simulink model "ddc_bpm_476_066"  (Simulink 7.8)
settings: Solver=ode45  StartTime=0.0  StopTime=2e-3  RelTol=1e-3
undefined symbols (not defined in the file): decim_factor_poly_35, dt_sim, frev_476, Fs_adc, n_ch, n_ovs, R_fofb, R_sec, R_sec_cfir, R_sec_pfir, R_tbt, xlipgetpartsetting
libraries: xbsIndex_r4 x1408, simulink x7
(part 9 of 11)

== system ddc_bpm_476_066/TBT_amp/TBT_amp0/TBT_poly_decim ==
  Q_in : Inport
  I_in : Inport  Port=2
  ch_in : Inport  Port=3
  Register1 : xbsIndex_r4/Register  init=0  rst=off  en=on  dbl_ovrd=off  block_type=register
  Register2 : xbsIndex_r4/Register  init=0  rst=off  en=off  dbl_ovrd=off  block_type=register
  Register3 : xbsIndex_r4/Register  init=0  rst=off  en=on  dbl_ovrd=off  block_type=register
  Register6 : xbsIndex_r4/Register  init=0  rst=off  en=off  dbl_ovrd=off  block_type=register
  Reinterpret : xbsIndex_r4/Reinterpret  force_arith_type=on  arith_type="Signed  (2's comp)"  force_bin_pt=on  bin_pt=23  block_type=reinterpret
      settings: block_version=10.1
  Reinterpret1 : xbsIndex_r4/Reinterpret  force_arith_type=on  arith_type="Signed  (2's comp)"  force_bin_pt=on  bin_pt=23  block_type=reinterpret
      settings: block_version=10.1
  ST3 : Subsystem
  Scope : Scope
      settings: YMin=1  YMax=1  SaveName=ScopeData4
  TBT_poly : xbsIndex_r4/FIR Compiler 6.3   coefficientvector=Hpoly_35.Numerator  coefficient_sets=1  coefficient_reload=off  filter_type=Decimation  rate_change_type=Integer  interpolation_rate=1  decimation_rate=decim_factor_poly_35  zero_pack_factor=1  channel_sequence=Basic  number_channels=2  pattern_list='P4-0,P4-1,P4-2,P4-3,P4-4'  number_paths=2  ratespecification=Maximum_Possible  sampleperiod=1  hardwareoversamplingrate=1  coefficient_sign=Signed  quantization=Quantize_Only  coefficient_width=16  bestprecision=on  coefficient_fractional_bits=20  coefficient_structure=Inferred  output_rounding_mode=Convergent_Rounding_to_Even  output_width=25  filter_architecture=Systolic_Multiply_Accumulate  optimization_goal=Area  data_buffer_type=Automatic  coefficient_buffer_type=Automatic  input_buffer_type=Automatic  output_buffer_type=Automatic  preference_for_other_storage=Automatic  multi_column_support=Automatic  columnconfig='13'  inter_column_pipe_length=4  data_has_tlast=Not_Required  m_data_has_tready=off  s_data_has_fifo=off  s_data_has_tuser=Chan_ID_Field  m_data_has_tuser=Chan_ID_Field  s_config_sync_mode=On_Vector  s_config_method=Single  num_reload_slots=1  has_aclken=off  has_aresetn=off  infoeditControl=ARESETn must be asserted for a minmum of 2 cycles  trim_axipin_name=on  passband_min=0.0  passband_max=0.5  stopband_min=0.5  stopband_max=1.0  filter_selection=1  gui_behaviour=Sysgen_GUI  data_sign=Signed  data_width=16  data_fractional_bits=0  data_tuser_width=1  wrapper_available=true  ip_wrap_arbitrary_binary_point=true  simulation_type=external_xfix  simulation_model=firv6_3_CModel:firv6_3_cmodel  ip_name=FIR Compiler  ip_version=6.3  dsptool_ready=true  ipcore_usecache=true  ipcore_useipmodelcache=true  ipcore_xco_need_fpga_part=true  port_translation_map={ 'aclken' => 'en', 'aresetn' => 'rst' }  run_core_at_system_period=true  ipcore_fpga_part=xlipgetpartsetting(gcb, {'virtex6', 'xc6vlx75t', '-3', 'ff784'})  block_type=fir_compiler_v6_3
      settings: infoedit=Maximum Possible : Maximizes oversampling rate. Abstracted input handshake (no s_data_tvalid) and automatic rate propagation.<br>Hardware Oversampling Rate : Specifies oversampling rate relative to the input sample period. Abstracted input handshake (no s_data_tvalid) and automatic rate propagation.<br>Sample Period : Specifies absolute oversampling rate. No input handshake abstraction (exposes s_data_tvalid) and no rate propagation.
  TDDM_TBT : Subsystem
  Terminator : Terminator
  Trunc : Subsystem
  Trunc1 : Subsystem
  tbt_decim_ch01_incorrect_o : xbsIndex_r4/Gateway Out  inherit_from_input=on  hdl_port=on  timing_constraint=Data Rate  locs_specified=off  LOCs={}  UseAsDAC=off  DACChannel='1'  block_type=gatewayout
      settings: infoedit="Gateway out block.  Converts Xilinx fixed-point or floating-point type inputs into ouputs of type Simulink integer, single, double, or fixed point.<br><br>Hardware notes:  In hardware these blocks become top level output ports or are discarded, depending on how they are configured."
  tbt_decim_ch0_i_o : xbsIndex_r4/Gateway Out  inherit_from_input=on  hdl_port=on  timing_constraint=Data Rate  locs_specified=off  LOCs={}  UseAsDAC=off  DACChannel='1'  block_type=gatewayout
      settings: infoedit="Gateway out block.  Converts Xilinx fixed-point or floating-point type inputs into ouputs of type Simulink integer, single, double, or fixed point.<br><br>Hardware notes:  In hardware these blocks become top level output ports or are discarded, depending on how they are configured."
  tbt_decim_ch0_q_o : xbsIndex_r4/Gateway Out  inherit_from_input=on  hdl_port=on  timing_constraint=Data Rate  locs_specified=off  LOCs={}  UseAsDAC=off  DACChannel='1'  block_type=gatewayout
      settings: infoedit="Gateway out block.  Converts Xilinx fixed-point or floating-point type inputs into ouputs of type Simulink integer, single, double, or fixed point.<br><br>Hardware notes:  In hardware these blocks become top level output ports or are discarded, depending on how they are configured."
  tbt_decim_ch1_i_o : xbsIndex_r4/Gateway Out  inherit_from_input=on  hdl_port=on  timing_constraint=Data Rate  locs_specified=off  LOCs={}  UseAsDAC=off  DACChannel='1'  block_type=gatewayout
      settings: infoedit="Gateway out block.  Converts Xilinx fixed-point or floating-point type inputs into ouputs of type Simulink integer, single, double, or fixed point.<br><br>Hardware notes:  In hardware these blocks become top level output ports or are discarded, depending on how they are configured."
  tbt_decim_ch1_q_o : xbsIndex_r4/Gateway Out  inherit_from_input=on  hdl_port=on  timing_constraint=Data Rate  locs_specified=off  LOCs={}  UseAsDAC=off  DACChannel='1'  block_type=gatewayout
      settings: infoedit="Gateway out block.  Converts Xilinx fixed-point or floating-point type inputs into ouputs of type Simulink integer, single, double, or fixed point.<br><br>Hardware notes:  In hardware these blocks become top level output ports or are discarded, depending on how they are configured."
  tbt_poly_i_scope : Scope  NumInputPorts=2
      settings: TimeRange=0.00011214  YMin=-0.1~-1.5  YMax=1~1.5  SaveName=ScopeData15  MaxDataPoints=1000000  SampleInput=on
  tbt_poly_q_scope : Scope  NumInputPorts=2
      settings: TimeRange=0.00011214  YMin=0.00109935~-0.000380039  YMax=0.00109935~-0.000380039  SaveName=ScopeData18  MaxDataPoints=1000000  SampleInput=on
  Q_out : Outport
  I_out : Outport  Port=2
  valid_out : Outport  Port=3
  ch_out : Outport  Port=4
  wires:
  Q_in/1 -> TBT_poly/2
  TBT_poly/4 -> Reinterpret/1
  TBT_poly/5 -> Reinterpret1/1
  I_in/1 -> TBT_poly/3
  TBT_poly/1 -> Terminator/1
  TBT_poly/3 -> Register2/1
  ch_in/1 -> ST3/1(In), TBT_poly/1
  [tbt_poly_q_out] -> Trunc/1(din)
  [tbt_poly_ch_out] -> TDDM_TBT/3(tbt_ch_in)
  [tbt_poly_i_out] -> Trunc1/1(din)
  Trunc/1(dout) -> TDDM_TBT/1(tbt_q_in)
  Trunc1/1(dout) -> TDDM_TBT/2(tbt_i_in)
  tbt_decim_ch0_q_o/1 -> tbt_poly_q_scope/1
  tbt_decim_ch1_q_o/1 -> tbt_poly_q_scope/2
  TDDM_TBT/1(poly35_ch0_q_out) -> tbt_decim_ch0_q_o/1
  TDDM_TBT/2(poly35_ch1_q_out) -> tbt_decim_ch1_q_o/1
  tbt_decim_ch0_i_o/1 -> tbt_poly_i_scope/1
  tbt_decim_ch1_i_o/1 -> tbt_poly_i_scope/2
  TDDM_TBT/3(poly35_ch0_i_out) -> tbt_decim_ch0_i_o/1
  TDDM_TBT/4(poly35_ch1_i_out) -> tbt_decim_ch1_i_o/1
  Register2/1 -> ch_out/1, [tbt_poly_ch_out]
  TBT_poly/2 -> Register6/1, Register1/2, Register3/2
  Register6/1 -> valid_out/1
  Reinterpret/1 -> Register1/1
  Register1/1 -> Q_out/1, [tbt_poly_q_out]
  Register3/1 -> I_out/1, [tbt_poly_i_out]
  Reinterpret1/1 -> Register3/1
  tbt_decim_ch01_incorrect_o/1 -> Scope/1
  TBT_poly/6 -> tbt_decim_ch01_incorrect_o/1

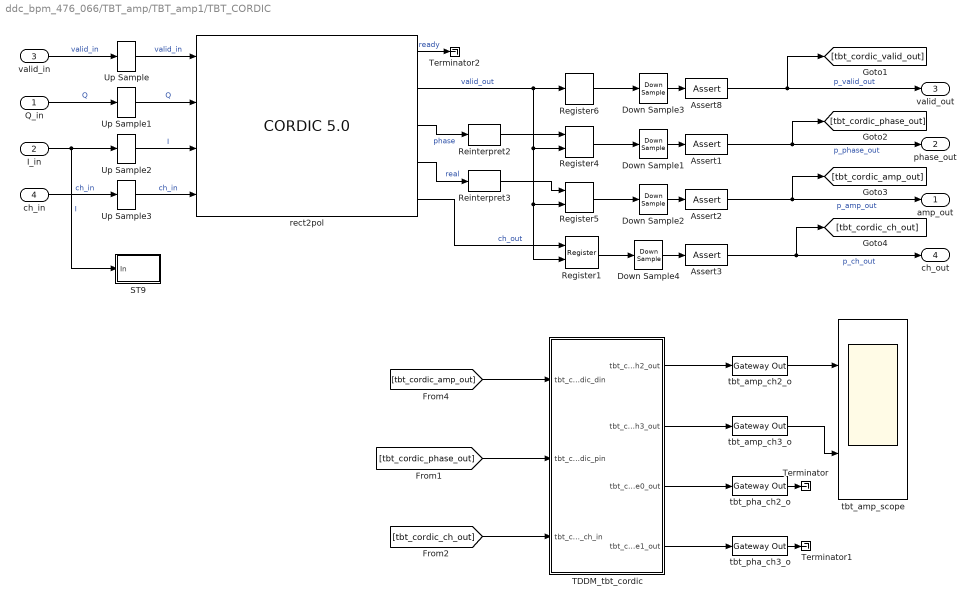
== system ddc_bpm_476_066/TBT_amp/TBT_amp1/TBT_CORDIC ==
  Q_in : Inport
  I_in : Inport  Port=2
  valid_in : Inport  Port=3
  ch_in : Inport  Port=4
  Assert{1..3,8} (4 alike) : xbsIndex_r4/Assert  assert_type=off  type_source=Explicitly  gui_display_data_type=Fixed-point  arith_type="Signed  (2's comp)"  n_bits=16  bin_pt=14  preci_type=Single  exp_width=8  frac_width=24  assert_rate=on  rate_source=Explicitly  period=(1/Fs_adc/n_ovs)*decim_factor_poly_35  output_port=on  block_type=assert
  Down Sample{1..4} (4 alike) : xbsIndex_r4/Down Sample  sample_ratio=decim_factor_poly_35  sample_phase="Last Value of Frame  (most efficient)"  en=off  latency=1  dbl_ovrd=off  block_type=dsamp
  Register1 : xbsIndex_r4/Register  init=0  rst=off  en=on  dbl_ovrd=off  block_type=register
  Register4 : xbsIndex_r4/Register  init=0  rst=off  en=on  dbl_ovrd=off  block_type=register
  Register5 : xbsIndex_r4/Register  init=0  rst=off  en=on  dbl_ovrd=off  block_type=register
  Register6 : xbsIndex_r4/Register  init=0  rst=off  en=off  dbl_ovrd=off  block_type=register
  Reinterpret2 : xbsIndex_r4/Reinterpret  force_arith_type=off  arith_type=Unsigned  force_bin_pt=off  bin_pt=18  block_type=reinterpret
  Reinterpret3 : xbsIndex_r4/Reinterpret  force_arith_type=off  arith_type=Unsigned  force_bin_pt=off  bin_pt=19  block_type=reinterpret
  ST9 : Subsystem
  TDDM_tbt_cordic : Subsystem
  Terminator : Terminator
  Terminator1 : Terminator
  Terminator2 : Terminator
  Up Sample : xbsIndex_r4/Up Sample  sample_ratio=R_tbt  copy_samples=off  en=off  latency=0  dbl_ovrd=off  block_type=usamp
  Up Sample1 : xbsIndex_r4/Up Sample  sample_ratio=R_tbt  copy_samples=on  en=off  latency=0  dbl_ovrd=off  block_type=usamp
  Up Sample2 : xbsIndex_r4/Up Sample  sample_ratio=R_tbt  copy_samples=on  en=off  latency=0  dbl_ovrd=off  block_type=usamp
  Up Sample3 : xbsIndex_r4/Up Sample  sample_ratio=R_tbt  copy_samples=on  en=off  latency=0  dbl_ovrd=off  block_type=usamp
  rect2pol : xbsIndex_r4/CORDIC 5.0   functional_selection=Translate  architectural_configuration=Word_Serial  pipelining_mode=Optimal  data_format=SignedFraction  phase_format=Radians  input_width=25  output_width=24  round_mode=Nearest_Even  iterations=0  precision=0  compensation_scaling=Embedded_Multiplier  coarse_rotation=on  aclken=off  aresetn=off  out_tready=off  cartesian_has_tuser=on  cartesian_has_tlast=off  cartesian_tuser_width=1  phase_has_tuser=off  phase_has_tlast=off  phase_tuser_width=1  out_tlast_behv=Null  flow_control=NonBlocking  optimize_goal=Resources  trim_axipin_name=on  ip_name=CORDIC  ip_version=5.0  dsptool_ready=true  ipcore_usecache=true  ipcore_useipmodelcache=true  wrapper_available=true  port_translation_map={ 'aclken' => 'en', 'aresetn' => 'rst' }  block_type=cordic_v5_0
      settings: infoedit=CORDIC 5.0
  tbt_amp_ch2_o : xbsIndex_r4/Gateway Out  inherit_from_input=on  hdl_port=on  timing_constraint=Data Rate  locs_specified=off  LOCs={}  UseAsDAC=off  DACChannel='1'  block_type=gatewayout
      settings: infoedit="Gateway out block.  Converts Xilinx fixed-point or floating-point type inputs into ouputs of type Simulink integer, single, double, or fixed point.<br><br>Hardware notes:  In hardware these blocks become top level output ports or are discarded, depending on how they are configured."
  tbt_amp_ch3_o : xbsIndex_r4/Gateway Out  inherit_from_input=on  hdl_port=on  timing_constraint=Data Rate  locs_specified=off  LOCs={}  UseAsDAC=off  DACChannel='1'  block_type=gatewayout
      settings: infoedit="Gateway out block.  Converts Xilinx fixed-point or floating-point type inputs into ouputs of type Simulink integer, single, double, or fixed point.<br><br>Hardware notes:  In hardware these blocks become top level output ports or are discarded, depending on how they are configured."
  tbt_amp_scope : Scope  NumInputPorts=2
      settings: TimeRange=0.00011214  YMin=0.109899~0.0274758  YMax=0.109899~0.0274758  SaveName=ScopeData19  MaxDataPoints=1000000  SampleInput=on
  tbt_pha_ch2_o : xbsIndex_r4/Gateway Out  inherit_from_input=on  hdl_port=on  timing_constraint=Data Rate  locs_specified=off  LOCs={}  UseAsDAC=off  DACChannel='1'  block_type=gatewayout
      settings: infoedit="Gateway out block.  Converts Xilinx fixed-point or floating-point type inputs into ouputs of type Simulink integer, single, double, or fixed point.<br><br>Hardware notes:  In hardware these blocks become top level output ports or are discarded, depending on how they are configured."
  tbt_pha_ch3_o : xbsIndex_r4/Gateway Out  inherit_from_input=off  hdl_port=on  timing_constraint=Data Rate  locs_specified=off  LOCs={}  UseAsDAC=off  DACChannel='1'  block_type=gatewayout
      settings: infoedit="Gateway out block.  Converts Xilinx fixed-point or floating-point type inputs into ouputs of type Simulink integer, single, double, or fixed point.<br><br>Hardware notes:  In hardware these blocks become top level output ports or are discarded, depending on how they are configured."
  amp_out : Outport
  phase_out : Outport  Port=2
  valid_out : Outport  Port=3
  ch_out : Outport  Port=4
  wires:
  [tbt_cordic_amp_out] -> TDDM_tbt_cordic/1(tbt_cordic_din)
  [tbt_cordic_ch_out] -> TDDM_tbt_cordic/3(tbt_cordic_ch_in)
  tbt_amp_ch2_o/1 -> tbt_amp_scope/1
  tbt_amp_ch3_o/1 -> tbt_amp_scope/2
  TDDM_tbt_cordic/1(tbt_cordic_ch2_out) -> tbt_amp_ch2_o/1
  TDDM_tbt_cordic/2(tbt_cordic_ch3_out) -> tbt_amp_ch3_o/1
  TDDM_tbt_cordic/3(tbt_cordic_phase0_out) -> tbt_pha_ch2_o/1
  TDDM_tbt_cordic/4(tbt_cordic_phase1_out) -> tbt_pha_ch3_o/1
  tbt_pha_ch2_o/1 -> Terminator/1
  tbt_pha_ch3_o/1 -> Terminator1/1
  [tbt_cordic_phase_out] -> TDDM_tbt_cordic/2(tbt_cordic_pin)
  Register4/1 -> Down Sample1/1
  Register5/1 -> Down Sample2/1
  Register6/1 -> Down Sample3/1
  Reinterpret2/1 -> Register4/1
  Reinterpret3/1 -> Register5/1
  valid_in/1 -> Up Sample/1  "valid_in"
  Q_in/1 -> Up Sample1/1  "Q"
  I_in/1 -> ST9/1(In), Up Sample2/1  "I"
  ch_in/1 -> Up Sample3/1  "ch_in"
  Register1/1 -> Down Sample4/1
  rect2pol/2 -> Register6/1, Register4/2, Register5/2, Register1/2  "valid_out"
  rect2pol/3 -> Reinterpret2/1  "phase"
  rect2pol/4 -> Reinterpret3/1  "real"
  rect2pol/5 -> Register1/1  "ch_out"
  rect2pol/1 -> Terminator2/1  "ready"
  Up Sample/1 -> rect2pol/1  "valid_in"
  Up Sample1/1 -> rect2pol/2  "Q"
  Up Sample2/1 -> rect2pol/3  "I"
  Up Sample3/1 -> rect2pol/4  "ch_in"
  Down Sample3/1 -> Assert8/1
  Assert8/1 -> valid_out/1, [tbt_cordic_valid_out]  "p_valid_out"
  Down Sample1/1 -> Assert1/1
  Down Sample2/1 -> Assert2/1
  Down Sample4/1 -> Assert3/1
  Assert1/1 -> phase_out/1, [tbt_cordic_phase_out]  "p_phase_out"
  Assert2/1 -> amp_out/1, [tbt_cordic_amp_out]  "p_amp_out"
  Assert3/1 -> ch_out/1, [tbt_cordic_ch_out]  "p_ch_out"

== system ddc_bpm_476_066/TBT_amp/TBT_amp1/TBT_poly_decim ==
  note: Introduced delays to avoid incorrect signal on the output
  Q_in : Inport
  I_in : Inport  Port=2
  ch_in : Inport  Port=3
  Register1 : xbsIndex_r4/Register  init=0  rst=off  en=on  dbl_ovrd=off  block_type=register
  Register2 : xbsIndex_r4/Register  init=0  rst=off  en=off  dbl_ovrd=off  block_type=register
  Register3 : xbsIndex_r4/Register  init=0  rst=off  en=on  dbl_ovrd=off  block_type=register
  Register6 : xbsIndex_r4/Register  init=0  rst=off  en=off  dbl_ovrd=off  block_type=register
  Reinterpret : xbsIndex_r4/Reinterpret  force_arith_type=on  arith_type="Signed  (2's comp)"  force_bin_pt=on  bin_pt=23  block_type=reinterpret
      settings: block_version=10.1
  Reinterpret1 : xbsIndex_r4/Reinterpret  force_arith_type=on  arith_type="Signed  (2's comp)"  force_bin_pt=on  bin_pt=23  block_type=reinterpret
      settings: block_version=10.1
  Scope : Scope
      settings: YMin=0.95  YMax=1.05  SaveName=ScopeData5
  TBT_poly : xbsIndex_r4/FIR Compiler 6.3   coefficientvector=Hpoly_35.Numerator  coefficient_sets=1  coefficient_reload=off  filter_type=Decimation  rate_change_type=Integer  interpolation_rate=1  decimation_rate=decim_factor_poly_35  zero_pack_factor=1  channel_sequence=Basic  number_channels=2  pattern_list='P4-0,P4-1,P4-2,P4-3,P4-4'  number_paths=2  ratespecification=Maximum_Possible  sampleperiod=1  hardwareoversamplingrate=2  coefficient_sign=Signed  quantization=Quantize_Only  coefficient_width=16  bestprecision=on  coefficient_fractional_bits=20  coefficient_structure=Inferred  output_rounding_mode=Convergent_Rounding_to_Even  output_width=25  filter_architecture=Systolic_Multiply_Accumulate  optimization_goal=Area  data_buffer_type=Automatic  coefficient_buffer_type=Automatic  input_buffer_type=Automatic  output_buffer_type=Automatic  preference_for_other_storage=Automatic  multi_column_support=Automatic  columnconfig='13'  inter_column_pipe_length=4  data_has_tlast=Not_Required  m_data_has_tready=off  s_data_has_fifo=off  s_data_has_tuser=Chan_ID_Field  m_data_has_tuser=Chan_ID_Field  s_config_sync_mode=On_Vector  s_config_method=Single  num_reload_slots=1  has_aclken=off  has_aresetn=off  infoeditControl=ARESETn must be asserted for a minmum of 2 cycles  trim_axipin_name=on  passband_min=0.0  passband_max=0.5  stopband_min=0.5  stopband_max=1.0  filter_selection=1  gui_behaviour=Sysgen_GUI  data_sign=Signed  data_width=16  data_fractional_bits=0  data_tuser_width=1  wrapper_available=true  ip_wrap_arbitrary_binary_point=true  simulation_type=external_xfix  simulation_model=firv6_3_CModel:firv6_3_cmodel  ip_name=FIR Compiler  ip_version=6.3  dsptool_ready=true  ipcore_usecache=true  ipcore_useipmodelcache=true  ipcore_xco_need_fpga_part=true  port_translation_map={ 'aclken' => 'en', 'aresetn' => 'rst' }  run_core_at_system_period=true  ipcore_fpga_part=xlipgetpartsetting(gcb, {'virtex6', 'xc6vlx75t', '-3', 'ff784'})  block_type=fir_compiler_v6_3
      settings: infoedit=Maximum Possible : Maximizes oversampling rate. Abstracted input handshake (no s_data_tvalid) and automatic rate propagation.<br>Hardware Oversampling Rate : Specifies oversampling rate relative to the input sample period. Abstracted input handshake (no s_data_tvalid) and automatic rate propagation.<br>Sample Period : Specifies absolute oversampling rate. No input handshake abstraction (exposes s_data_tvalid) and no rate propagation.
  TDDM_TBT : Subsystem
  Terminator : Terminator
  Trunc : Subsystem
  Trunc1 : Subsystem
  tbt_decim_ch23_incorrect_o : xbsIndex_r4/Gateway Out  inherit_from_input=on  hdl_port=on  timing_constraint=Data Rate  locs_specified=off  LOCs={}  UseAsDAC=off  DACChannel='1'  block_type=gatewayout
      settings: infoedit="Gateway out block.  Converts Xilinx fixed-point or floating-point type inputs into ouputs of type Simulink integer, single, double, or fixed point.<br><br>Hardware notes:  In hardware these blocks become top level output ports or are discarded, depending on how they are configured."
  tbt_decim_ch2_i_o : xbsIndex_r4/Gateway Out  inherit_from_input=on  hdl_port=on  timing_constraint=Data Rate  locs_specified=off  LOCs={}  UseAsDAC=off  DACChannel='1'  block_type=gatewayout
      settings: infoedit="Gateway out block.  Converts Xilinx fixed-point or floating-point type inputs into ouputs of type Simulink integer, single, double, or fixed point.<br><br>Hardware notes:  In hardware these blocks become top level output ports or are discarded, depending on how they are configured."
  tbt_decim_ch2_q_o : xbsIndex_r4/Gateway Out  inherit_from_input=on  hdl_port=on  timing_constraint=Data Rate  locs_specified=off  LOCs={}  UseAsDAC=off  DACChannel='1'  block_type=gatewayout
      settings: infoedit="Gateway out block.  Converts Xilinx fixed-point or floating-point type inputs into ouputs of type Simulink integer, single, double, or fixed point.<br><br>Hardware notes:  In hardware these blocks become top level output ports or are discarded, depending on how they are configured."
  tbt_decim_ch3_i_o : xbsIndex_r4/Gateway Out  inherit_from_input=on  hdl_port=on  timing_constraint=Data Rate  locs_specified=off  LOCs={}  UseAsDAC=off  DACChannel='1'  block_type=gatewayout
      settings: infoedit="Gateway out block.  Converts Xilinx fixed-point or floating-point type inputs into ouputs of type Simulink integer, single, double, or fixed point.<br><br>Hardware notes:  In hardware these blocks become top level output ports or are discarded, depending on how they are configured."
  tbt_decim_ch3_q_o : xbsIndex_r4/Gateway Out  inherit_from_input=on  hdl_port=on  timing_constraint=Data Rate  locs_specified=off  LOCs={}  UseAsDAC=off  DACChannel='1'  block_type=gatewayout
      settings: infoedit="Gateway out block.  Converts Xilinx fixed-point or floating-point type inputs into ouputs of type Simulink integer, single, double, or fixed point.<br><br>Hardware notes:  In hardware these blocks become top level output ports or are discarded, depending on how they are configured."
  tbt_poly_i_scope : Scope  NumInputPorts=2
      settings: TimeRange=0.00011214  YMin=-0.1~-1.5  YMax=1~1.5  SaveName=ScopeData15  MaxDataPoints=1000000  SampleInput=on
  tbt_poly_q_scope : Scope  NumInputPorts=2
      settings: TimeRange=0.00011214  YMin=-0.1~-1.5  YMax=1~1.5  SaveName=ScopeData18  MaxDataPoints=1000000  SampleInput=on
  Q_out : Outport
  I_out : Outport  Port=2
  valid_out : Outport  Port=3
  ch_out : Outport  Port=4
  wires:
  Q_in/1 -> TBT_poly/2
  TBT_poly/4 -> Reinterpret/1
  TBT_poly/5 -> Reinterpret1/1
  I_in/1 -> TBT_poly/3
  TBT_poly/1 -> Terminator/1
  ch_in/1 -> TBT_poly/1
  [tbt_poly_q_out] -> Trunc/1(din)
  [tbt_poly_ch_out] -> TDDM_TBT/3(tbt_ch_in)
  [tbt_poly_i_out] -> Trunc1/1(din)
  Trunc/1(dout) -> TDDM_TBT/1(tbt_q_in)
  Trunc1/1(dout) -> TDDM_TBT/2(tbt_i_in)
  tbt_decim_ch2_q_o/1 -> tbt_poly_q_scope/1
  tbt_decim_ch3_q_o/1 -> tbt_poly_q_scope/2
  TDDM_TBT/1(poly35_ch2_q_out) -> tbt_decim_ch2_q_o/1
  TDDM_TBT/2(poly35_ch3_q_out) -> tbt_decim_ch3_q_o/1
  tbt_decim_ch2_i_o/1 -> tbt_poly_i_scope/1
  tbt_decim_ch3_i_o/1 -> tbt_poly_i_scope/2
  TDDM_TBT/3(poly35_ch2_i_out) -> tbt_decim_ch2_i_o/1
  TDDM_TBT/4(poly35_ch3_i_out) -> tbt_decim_ch3_i_o/1
  TBT_poly/2 -> Register6/1, Register3/2, Register1/2
  Register6/1 -> valid_out/1
  TBT_poly/3 -> Register2/1
  Register2/1 -> ch_out/1, [tbt_poly_ch_out]
  Reinterpret/1 -> Register1/1
  Reinterpret1/1 -> Register3/1
  Register1/1 -> Q_out/1, [tbt_poly_q_out]
  Register3/1 -> I_out/1, [tbt_poly_i_out]
  tbt_decim_ch23_incorrect_o/1 -> Scope/1
  TBT_poly/6 -> tbt_decim_ch23_incorrect_o/1

== system ddc_bpm_476_066/TBT_amp/TDDM_tbt_amp_4ch/TDDM_tbt_amp0 ==
  din : Inport
  ch_in : Inport  Port=2
  Constant : xbsIndex_r4/Constant  const=1  gui_display_data_type=Fixed-point  arith_type=Unsigned  n_bits=1  bin_pt=0  preci_type=Single  exp_width=8  frac_width=24  explicit_period=off  period=1  equ=P=C  opselect=C  inp2=PCIN>>17  opr=+  inp1=P  carry=CIN  dbl_ovrd=off  block_type=constant
  Constant1 : xbsIndex_r4/Constant  const=0  gui_display_data_type=Fixed-point  arith_type=Unsigned  n_bits=1  bin_pt=0  preci_type=Single  exp_width=8  frac_width=24  explicit_period=off  period=1  equ=P=C  opselect=C  inp2=PCIN>>17  opr=+  inp1=P  carry=CIN  dbl_ovrd=off  block_type=constant
  Delay : xbsIndex_r4/Delay  rst=off  infoeditControl=Selection of Reset will increase slice count due to use of real FFs and instead of SRLs  en=off  latency=3  dbl_ovrd=off  reg_retiming=off  block_type=delay
  Down Sample1 : xbsIndex_r4/Down Sample  sample_ratio=n_ch/n_ovs  sample_phase="Last Value of Frame  (most efficient)"  en=off  latency=1  dbl_ovrd=off  block_type=dsamp
  Down Sample2 : xbsIndex_r4/Down Sample  sample_ratio=n_ch/n_ovs  sample_phase="Last Value of Frame  (most efficient)"  en=off  latency=1  dbl_ovrd=off  block_type=dsamp
  Register : xbsIndex_r4/Register  init=0  rst=off  en=on  dbl_ovrd=off  block_type=register
  Register1 : xbsIndex_r4/Register  init=0  rst=off  en=on  dbl_ovrd=off  block_type=register
  Relational : xbsIndex_r4/Relational  mode=a=b  en=off  latency=1  dbl_ovrd=off  block_type=relational
  Relational1 : xbsIndex_r4/Relational  mode=a=b  en=off  latency=1  dbl_ovrd=off  block_type=relational
  dout_ch0 : Outport
  dout_ch1 : Outport  Port=2
  ch_out : Outport  Port=3
  wires:
  Constant/1 -> Relational/2
  Constant1/1 -> Relational1/2
  Relational/1 -> Register/2
  Relational1/1 -> Register1/2
  din/1 -> Register/1, Register1/1
  Register/1 -> Down Sample2/1
  ch_in/1 -> Relational/1, Relational1/1, Delay/1
  Register1/1 -> Down Sample1/1
  Down Sample2/1 -> dout_ch0/1
  Delay/1 -> ch_out/1
  Down Sample1/1 -> dout_ch1/1

== system ddc_bpm_476_066/TBT_amp/TDDM_tbt_amp_4ch/TDDM_tbt_amp1 ==
  din : Inport
  ch_in : Inport  Port=2
  Constant : xbsIndex_r4/Constant  const=1  gui_display_data_type=Fixed-point  arith_type=Unsigned  n_bits=1  bin_pt=0  preci_type=Single  exp_width=8  frac_width=24  explicit_period=off  period=1  equ=P=C  opselect=C  inp2=PCIN>>17  opr=+  inp1=P  carry=CIN  dbl_ovrd=off  block_type=constant
  Constant1 : xbsIndex_r4/Constant  const=0  gui_display_data_type=Fixed-point  arith_type=Unsigned  n_bits=1  bin_pt=0  preci_type=Single  exp_width=8  frac_width=24  explicit_period=off  period=1  equ=P=C  opselect=C  inp2=PCIN>>17  opr=+  inp1=P  carry=CIN  dbl_ovrd=off  block_type=constant
  Delay : xbsIndex_r4/Delay  rst=off  infoeditControl=Selection of Reset will increase slice count due to use of real FFs and instead of SRLs  en=off  latency=3  dbl_ovrd=off  reg_retiming=off  block_type=delay
  Down Sample1 : xbsIndex_r4/Down Sample  sample_ratio=n_ch/n_ovs  sample_phase="Last Value of Frame  (most efficient)"  en=off  latency=1  dbl_ovrd=off  block_type=dsamp
  Down Sample2 : xbsIndex_r4/Down Sample  sample_ratio=n_ch/n_ovs  sample_phase="Last Value of Frame  (most efficient)"  en=off  latency=1  dbl_ovrd=off  block_type=dsamp
  Register : xbsIndex_r4/Register  init=0  rst=off  en=on  dbl_ovrd=off  block_type=register
  Register1 : xbsIndex_r4/Register  init=0  rst=off  en=on  dbl_ovrd=off  block_type=register
  Relational : xbsIndex_r4/Relational  mode=a=b  en=off  latency=1  dbl_ovrd=off  block_type=relational
  Relational1 : xbsIndex_r4/Relational  mode=a=b  en=off  latency=1  dbl_ovrd=off  block_type=relational
  dout_ch0 : Outport
  dout_ch1 : Outport  Port=2
  ch_out : Outport  Port=3
  wires:
  Constant/1 -> Relational/2
  Constant1/1 -> Relational1/2
  Relational/1 -> Register/2
  Relational1/1 -> Register1/2
  din/1 -> Register/1, Register1/1
  Register/1 -> Down Sample2/1
  ch_in/1 -> Relational/1, Relational1/1, Delay/1
  Register1/1 -> Down Sample1/1
  Down Sample2/1 -> dout_ch0/1
  Delay/1 -> ch_out/1
  Down Sample1/1 -> dout_ch1/1

== system ddc_bpm_476_066/TDM_mix/TDM_mix_ch0_1/ST1 ==
  In : Inport
  Display : Display
  Sample Time : xbsIndex_r4/Sample Time  block_type=sampletime
      settings: infoedit="The Sample Time block reports the normalized sample period of its input.  A signal's normalized sample period is not equivalent to its Simulink absolute sample period.<br><br>Hardware notes: This block is implemented as a constant in hardware."
  X_monit1 : xbsIndex_r4/Gateway Out  inherit_from_input=on  hdl_port=off  timing_constraint=Data Rate  locs_specified=off  LOCs={}  UseAsDAC=off  DACChannel='1'  block_type=gatewayout
      settings: infoedit="Gateway out block.  Converts Xilinx fixed-point or floating-point type inputs into ouputs of type Simulink integer, single, double, or fixed point.<br><br>Hardware notes:  In hardware these blocks become top level output ports or are discarded, depending on how they are configured."
  wires:
  X_monit1/1 -> Display/1
  Sample Time/1 -> X_monit1/1
  In/1 -> Sample Time/1

== system ddc_bpm_476_066/TDM_mix/TDM_mix_ch0_1/ST2 ==
  In : Inport
  Display : Display
  Sample Time : xbsIndex_r4/Sample Time  block_type=sampletime
      settings: infoedit="The Sample Time block reports the normalized sample period of its input.  A signal's normalized sample period is not equivalent to its Simulink absolute sample period.<br><br>Hardware notes: This block is implemented as a constant in hardware."
  X_monit1 : xbsIndex_r4/Gateway Out  inherit_from_input=on  hdl_port=off  timing_constraint=Data Rate  locs_specified=off  LOCs={}  UseAsDAC=off  DACChannel='1'  block_type=gatewayout
      settings: infoedit="Gateway out block.  Converts Xilinx fixed-point or floating-point type inputs into ouputs of type Simulink integer, single, double, or fixed point.<br><br>Hardware notes:  In hardware these blocks become top level output ports or are discarded, depending on how they are configured."
  wires:
  X_monit1/1 -> Display/1
  Sample Time/1 -> X_monit1/1
  In/1 -> Sample Time/1

== system ddc_bpm_476_066/TDM_mix/TDM_mix_ch0_1/ST3 ==
  In : Inport
  Display : Display
  Sample Time : xbsIndex_r4/Sample Time  block_type=sampletime
      settings: infoedit="The Sample Time block reports the normalized sample period of its input.  A signal's normalized sample period is not equivalent to its Simulink absolute sample period.<br><br>Hardware notes: This block is implemented as a constant in hardware."
  X_monit1 : xbsIndex_r4/Gateway Out  inherit_from_input=on  hdl_port=off  timing_constraint=Data Rate  locs_specified=off  LOCs={}  UseAsDAC=off  DACChannel='1'  block_type=gatewayout
      settings: infoedit="Gateway out block.  Converts Xilinx fixed-point or floating-point type inputs into ouputs of type Simulink integer, single, double, or fixed point.<br><br>Hardware notes:  In hardware these blocks become top level output ports or are discarded, depending on how they are configured."
  wires:
  X_monit1/1 -> Display/1
  Sample Time/1 -> X_monit1/1
  In/1 -> Sample Time/1

== system ddc_bpm_476_066/TDM_mix/TDM_mix_ch0_1/ST5 ==
  In : Inport
  Display : Display
  Sample Time : xbsIndex_r4/Sample Time  block_type=sampletime
      settings: infoedit="The Sample Time block reports the normalized sample period of its input.  A signal's normalized sample period is not equivalent to its Simulink absolute sample period.<br><br>Hardware notes: This block is implemented as a constant in hardware."
  out : xbsIndex_r4/Gateway Out  inherit_from_input=on  hdl_port=off  timing_constraint=Data Rate  locs_specified=off  LOCs={}  UseAsDAC=off  DACChannel='1'  block_type=gatewayout
      settings: infoedit="Gateway out block.  Converts Xilinx fixed-point or floating-point type inputs into ouputs of type Simulink integer, single, double, or fixed point.<br><br>Hardware notes:  In hardware these blocks become top level output ports or are discarded, depending on how they are configured."
  wires:
  out/1 -> Display/1
  Sample Time/1 -> out/1
  In/1 -> Sample Time/1

== system ddc_bpm_476_066/TDM_mix/TDM_mix_ch0_2/ST1 ==
  In : Inport
  Display : Display
  Sample Time : xbsIndex_r4/Sample Time  block_type=sampletime
      settings: infoedit="The Sample Time block reports the normalized sample period of its input.  A signal's normalized sample period is not equivalent to its Simulink absolute sample period.<br><br>Hardware notes: This block is implemented as a constant in hardware."
  X_monit1 : xbsIndex_r4/Gateway Out  inherit_from_input=on  hdl_port=off  timing_constraint=Data Rate  locs_specified=off  LOCs={}  UseAsDAC=off  DACChannel='1'  block_type=gatewayout
      settings: infoedit="Gateway out block.  Converts Xilinx fixed-point or floating-point type inputs into ouputs of type Simulink integer, single, double, or fixed point.<br><br>Hardware notes:  In hardware these blocks become top level output ports or are discarded, depending on how they are configured."
  wires:
  X_monit1/1 -> Display/1
  Sample Time/1 -> X_monit1/1
  In/1 -> Sample Time/1

== system ddc_bpm_476_066/TDM_mix/TDM_mix_ch0_2/ST2 ==
  In : Inport
  Display : Display
  Sample Time : xbsIndex_r4/Sample Time  block_type=sampletime
      settings: infoedit="The Sample Time block reports the normalized sample period of its input.  A signal's normalized sample period is not equivalent to its Simulink absolute sample period.<br><br>Hardware notes: This block is implemented as a constant in hardware."
  X_monit1 : xbsIndex_r4/Gateway Out  inherit_from_input=on  hdl_port=off  timing_constraint=Data Rate  locs_specified=off  LOCs={}  UseAsDAC=off  DACChannel='1'  block_type=gatewayout
      settings: infoedit="Gateway out block.  Converts Xilinx fixed-point or floating-point type inputs into ouputs of type Simulink integer, single, double, or fixed point.<br><br>Hardware notes:  In hardware these blocks become top level output ports or are discarded, depending on how they are configured."
  wires:
  X_monit1/1 -> Display/1
  Sample Time/1 -> X_monit1/1
  In/1 -> Sample Time/1

== system ddc_bpm_476_066/TDM_mix/TDM_mix_ch0_2/ST3 ==
  In : Inport
  Display : Display
  Sample Time : xbsIndex_r4/Sample Time  block_type=sampletime
      settings: infoedit="The Sample Time block reports the normalized sample period of its input.  A signal's normalized sample period is not equivalent to its Simulink absolute sample period.<br><br>Hardware notes: This block is implemented as a constant in hardware."
  X_monit1 : xbsIndex_r4/Gateway Out  inherit_from_input=on  hdl_port=off  timing_constraint=Data Rate  locs_specified=off  LOCs={}  UseAsDAC=off  DACChannel='1'  block_type=gatewayout
      settings: infoedit="Gateway out block.  Converts Xilinx fixed-point or floating-point type inputs into ouputs of type Simulink integer, single, double, or fixed point.<br><br>Hardware notes:  In hardware these blocks become top level output ports or are discarded, depending on how they are configured."
  wires:
  X_monit1/1 -> Display/1
  Sample Time/1 -> X_monit1/1
  In/1 -> Sample Time/1

== system ddc_bpm_476_066/TDM_mix/TDM_mix_ch0_2/ST5 ==
  In : Inport
  Display : Display
  Sample Time : xbsIndex_r4/Sample Time  block_type=sampletime
      settings: infoedit="The Sample Time block reports the normalized sample period of its input.  A signal's normalized sample period is not equivalent to its Simulink absolute sample period.<br><br>Hardware notes: This block is implemented as a constant in hardware."
  out : xbsIndex_r4/Gateway Out  inherit_from_input=on  hdl_port=off  timing_constraint=Data Rate  locs_specified=off  LOCs={}  UseAsDAC=off  DACChannel='1'  block_type=gatewayout
      settings: infoedit="Gateway out block.  Converts Xilinx fixed-point or floating-point type inputs into ouputs of type Simulink integer, single, double, or fixed point.<br><br>Hardware notes:  In hardware these blocks become top level output ports or are discarded, depending on how they are configured."
  wires:
  out/1 -> Display/1
  Sample Time/1 -> out/1
  In/1 -> Sample Time/1

== system ddc_bpm_476_066/monit_pos_1/Cast1/format1 ==
  din : Inport
  Convert : xbsIndex_r4/Convert  gui_display_data_type=Fixed-point  arith_type="Signed  (2's comp)"  n_bits=25  bin_pt=24  float_type=Single  exp_bits=8  fraction_bits=24  quantization="Round  (unbiased: +/- Inf)"  overflow=Flag as error  en=off  latency=0  dbl_ovrd=off  pipeline=off  block_type=convert
  Reinterpret : xbsIndex_r4/Reinterpret  force_arith_type=on  arith_type="Signed  (2's comp)"  force_bin_pt=off  bin_pt=22  block_type=reinterpret
      settings: block_version=10.1
  dout : Outport
  wires:
  din/1 -> Reinterpret/1
  Reinterpret/1 -> Convert/1
  Convert/1 -> dout/1

== system ddc_bpm_476_066/monit_pos_1/TDDM_monit_pos_1_out/TDDM_monit_pos_1_out_int ==
  din : Inport
  ch_in : Inport  Port=2
  Constant : xbsIndex_r4/Constant  const=3  gui_display_data_type=Fixed-point  arith_type=Unsigned  n_bits=2  bin_pt=0  preci_type=Single  exp_width=8  frac_width=24  explicit_period=off  period=1  equ=P=C  opselect=C  inp2=PCIN>>17  opr=+  inp1=P  carry=CIN  dbl_ovrd=off  block_type=constant
  Constant1 : xbsIndex_r4/Constant  const=0  gui_display_data_type=Fixed-point  arith_type=Unsigned  n_bits=2  bin_pt=0  preci_type=Single  exp_width=8  frac_width=24  explicit_period=off  period=1  equ=P=C  opselect=C  inp2=PCIN>>17  opr=+  inp1=P  carry=CIN  dbl_ovrd=off  block_type=constant
  Constant3 : xbsIndex_r4/Constant  const=1  gui_display_data_type=Fixed-point  arith_type=Unsigned  n_bits=2  bin_pt=0  preci_type=Single  exp_width=8  frac_width=24  explicit_period=off  period=1  equ=P=C  opselect=C  inp2=PCIN>>17  opr=+  inp1=P  carry=CIN  dbl_ovrd=off  block_type=constant
  Constant4 : xbsIndex_r4/Constant  const=2  gui_display_data_type=Fixed-point  arith_type=Unsigned  n_bits=2  bin_pt=0  preci_type=Single  exp_width=8  frac_width=24  explicit_period=off  period=1  equ=P=C  opselect=C  inp2=PCIN>>17  opr=+  inp1=P  carry=CIN  dbl_ovrd=off  block_type=constant
  Delay : xbsIndex_r4/Delay  rst=off  infoeditControl=Selection of Reset will increase slice count due to use of real FFs and instead of SRLs  en=off  latency=3  dbl_ovrd=off  reg_retiming=off  block_type=delay
  Down Sample{1..4} (4 alike) : xbsIndex_r4/Down Sample  sample_ratio=n_ch  sample_phase="Last Value of Frame  (most efficient)"  en=off  latency=1  dbl_ovrd=off  block_type=dsamp
  Register{,1..3} (4 alike) : xbsIndex_r4/Register  init=0  rst=off  en=on  dbl_ovrd=off  block_type=register
  Relational{,1..3} (4 alike) : xbsIndex_r4/Relational  mode=a=b  en=off  latency=1  dbl_ovrd=off  block_type=relational
  dout_ch0 : Outport
  dout_ch1 : Outport  Port=2
  dout_ch2 : Outport  Port=3
  dout_ch3 : Outport  Port=4
  ch_out : Outport  Port=5
  wires:
  Constant/1 -> Relational/2
  Constant1/1 -> Relational1/2
  Constant3/1 -> Relational2/2
  Constant4/1 -> Relational3/2
  Relational/1 -> Register/2
  Relational1/1 -> Register1/2
  Relational2/1 -> Register2/2
  Relational3/1 -> Register3/2
  din/1 -> Register1/1, Register2/1, Register3/1, Register/1
  Register/1 -> Down Sample2/1
  ch_in/1 -> Relational/1, Relational1/1, Relational2/1, Relational3/1, Delay/1
  Register1/1 -> Down Sample1/1
  Register2/1 -> Down Sample3/1
  Register3/1 -> Down Sample4/1
  Down Sample2/1 -> dout_ch0/1
  Delay/1 -> ch_out/1
  Down Sample3/1 -> dout_ch2/1
  Down Sample1/1 -> dout_ch1/1
  Down Sample4/1 -> dout_ch3/1

== system ddc_bpm_476_066/FOFB_amp/fofb_amp0/FOFB_CORDIC/TDDM_tbt_cordic0 ==
  fofb_cordic_din : Inport
  fofb_cordic_pin : Inport  Port=2
  fofb_cordic_ch_in : Inport  Port=3
  TDDM_fofb_cordic0_int : Subsystem
  TDDM_tbt_cordic1 : Subsystem
  Terminator : Terminator
  Terminator1 : Terminator
  fofb_cordic_data0_out : Outport
  fofb_cordic_data1_out : Outport  Port=2
  fofb_cordic_phase0_out : Outport  Port=3
  fofb_cordic_phase1_out : Outport  Port=4
  wires:
  TDDM_fofb_cordic0_int/2(dout_ch1) -> fofb_cordic_data1_out/1
  fofb_cordic_din/1 -> TDDM_fofb_cordic0_int/1(din)
  fofb_cordic_ch_in/1 -> TDDM_fofb_cordic0_int/2(ch_in), TDDM_tbt_cordic1/2(ch_in)
  TDDM_fofb_cordic0_int/1(dout_ch0) -> fofb_cordic_data0_out/1
  TDDM_fofb_cordic0_int/3(ch_out) -> Terminator/1
  TDDM_tbt_cordic1/2(dout_ch1) -> fofb_cordic_phase1_out/1
  fofb_cordic_pin/1 -> TDDM_tbt_cordic1/1(din)
  TDDM_tbt_cordic1/1(dout_ch0) -> fofb_cordic_phase0_out/1
  TDDM_tbt_cordic1/3(ch_out) -> Terminator1/1

== system ddc_bpm_476_066/FOFB_amp/fofb_amp0/FOFB_amp/Reg ==
  din : Inport
  Convert : xbsIndex_r4/Convert  gui_display_data_type=Fixed-point  arith_type="Signed  (2's comp)"  n_bits=24  bin_pt=22  float_type=Single  exp_bits=8  fraction_bits=24  quantization="Round  (unbiased: +/- Inf)"  overflow=Flag as error  en=off  latency=0  dbl_ovrd=off  pipeline=off  block_type=convert
  Register : xbsIndex_r4/Register  init=0  rst=off  en=off  dbl_ovrd=off  block_type=register
      settings: xl_area=[0, 0, 0, 0, 0, 0, 0]  block_version=VER_STRING_GOES_HERE
  Reinterpret2 : xbsIndex_r4/Reinterpret  force_arith_type=on  arith_type="Signed  (2's comp)"  force_bin_pt=on  bin_pt=23  block_type=cast
      settings: block_version=VER_STRING_GOES_HERE
  dout : Outport
  wires:
  Register/1 -> dout/1
  din/1 -> Reinterpret2/1
  Reinterpret2/1 -> Convert/1
  Convert/1 -> Register/1

== system ddc_bpm_476_066/FOFB_amp/fofb_amp0/FOFB_amp/Reg1 ==
  din : Inport
  Convert : xbsIndex_r4/Convert  gui_display_data_type=Fixed-point  arith_type="Signed  (2's comp)"  n_bits=24  bin_pt=22  float_type=Single  exp_bits=8  fraction_bits=24  quantization="Round  (unbiased: +/- Inf)"  overflow=Flag as error  en=off  latency=0  dbl_ovrd=off  pipeline=off  block_type=convert
  Register : xbsIndex_r4/Register  init=0  rst=off  en=off  dbl_ovrd=off  block_type=register
      settings: xl_area=[0, 0, 0, 0, 0, 0, 0]  block_version=VER_STRING_GOES_HERE
  Reinterpret2 : xbsIndex_r4/Reinterpret  force_arith_type=on  arith_type="Signed  (2's comp)"  force_bin_pt=on  bin_pt=23  block_type=cast
      settings: block_version=VER_STRING_GOES_HERE
  dout : Outport
  wires:
  Register/1 -> dout/1
  din/1 -> Reinterpret2/1
  Reinterpret2/1 -> Convert/1
  Convert/1 -> Register/1

== system ddc_bpm_476_066/FOFB_amp/fofb_amp0/FOFB_amp/TDDM_fofb_cic0 ==
  fofb_q_in : Inport
  fofb_i_in : Inport  Port=2
  fofb_ch_in : Inport  Port=3
  TDDM_fofb_cic0_i : Subsystem
  TDDM_fofb_cic0_q : Subsystem
  Terminator : Terminator
  Terminator1 : Terminator
  cic_fofb_ch0_q_out : Outport
  cic_fofb_ch1_q_out : Outport  Port=2
  cic_fofb_ch0_i_out : Outport  Port=3
  cic_fofb_ch1_i_out : Outport  Port=4
  wires:
  fofb_q_in/1 -> TDDM_fofb_cic0_q/1(din)
  fofb_ch_in/1 -> TDDM_fofb_cic0_q/2(ch_in), TDDM_fofb_cic0_i/2(ch_in)
  fofb_i_in/1 -> TDDM_fofb_cic0_i/1(din)
  TDDM_fofb_cic0_q/1(dout_ch0) -> cic_fofb_ch0_q_out/1
  TDDM_fofb_cic0_q/2(dout_ch1) -> cic_fofb_ch1_q_out/1
  TDDM_fofb_cic0_i/2(dout_ch1) -> cic_fofb_ch1_i_out/1
  TDDM_fofb_cic0_i/1(dout_ch0) -> cic_fofb_ch0_i_out/1
  TDDM_fofb_cic0_i/3(ch_out) -> Terminator/1
  TDDM_fofb_cic0_q/3(ch_out) -> Terminator1/1

== system ddc_bpm_476_066/FOFB_amp/fofb_amp0/FOFB_amp/cic_fofb ==
  ch_in : Inport
  Q_in : Inport  Port=2
  I_in : Inport  Port=3
  Constant1 : xbsIndex_r4/Constant  const=0  gui_display_data_type=Fixed-point  arith_type=Unsigned  n_bits=2  bin_pt=0  preci_type=Single  exp_width=8  frac_width=24  explicit_period=off  period=1  equ=P=C  opselect=C  inp2=PCIN>>17  opr=+  inp1=P  carry=CIN  dbl_ovrd=off  block_type=constant
  Delay : xbsIndex_r4/Delay  rst=off  infoeditControl=Selection of Reset will increase slice count due to use of real FFs and instead of SRLs  en=off  latency=1  dbl_ovrd=off  reg_retiming=off  block_type=delay
  Gateway Out{1..6} (6 alike) : xbsIndex_r4/Gateway Out  inherit_from_input=on  hdl_port=off  timing_constraint=Data Rate  locs_specified=off  LOCs={}  UseAsDAC=off  DACChannel='1'  block_type=gatewayout
      settings: infoedit="Gateway out block.  Converts Xilinx fixed-point or floating-point type inputs into ouputs of type Simulink integer, single, double, or fixed point.<br><br>Hardware notes:  In hardware these blocks become top level output ports or are discarded, depending on how they are configured."
  Reg : Subsystem
  Reg1 : Subsystem
  Relational2 : xbsIndex_r4/Relational  mode=a=b  en=off  latency=1  dbl_ovrd=off  block_type=relational
  Terminator{,1..3,5..9,11} (10 alike) : Terminator
  cic_fofb_i : xbsIndex_r4/CIC Compiler 3.0   filter_type=Decimation  number_of_stages=3  differential_delay=2  number_of_channels=2  sample_rate_changes=Fixed  fixed_or_initial_rate=R_fofb  minimum_rate=1000  maximum_rate=1000  ratespecification=Maximum_Possible  sampleperiod=1  hardwareoversamplingrate=1  quantization=Full_Precision  output_data_width=51  use_xtreme_dsp_slice=on  use_streaming_interface=on  has_aclken=off  has_aresetn=off  has_dout_tready=off  trim_axipin_name=on  gui_behaviour=Sysgen_GUI  input_data_width=18  ip_name=CIC Compiler  ip_version=3.0  dsptool_ready=true  wrapper_available=true  port_translation_map={ 'aclken' => 'en', 'aresetn' => 'rst' }  ipcore_xco_need_fpga_part=true  ipcore_fpga_part=xlipgetpartsetting(gcb, {'virtex7', 'xc7v1500t', '-2', 'fhg1157'})  ipcore_verbose=false  block_type=cic_compiler_v3_0
  cic_fofb_q : xbsIndex_r4/CIC Compiler 3.0   filter_type=Decimation  number_of_stages=3  differential_delay=2  number_of_channels=2  sample_rate_changes=Fixed  fixed_or_initial_rate=R_fofb  minimum_rate=1000  maximum_rate=1000  ratespecification=Maximum_Possible  sampleperiod=1  hardwareoversamplingrate=1  quantization=Full_Precision  output_data_width=51  use_xtreme_dsp_slice=on  use_streaming_interface=on  has_aclken=off  has_aresetn=off  has_dout_tready=off  trim_axipin_name=on  gui_behaviour=Sysgen_GUI  input_data_width=18  ip_name=CIC Compiler  ip_version=3.0  dsptool_ready=true  wrapper_available=true  port_translation_map={ 'aclken' => 'en', 'aresetn' => 'rst' }  ipcore_xco_need_fpga_part=true  ipcore_fpga_part=xlipgetpartsetting(gcb, {'virtex7', 'xc7v1500t', '-2', 'fhg1157'})  ipcore_verbose=false  block_type=cic_compiler_v3_0
  cic_fofb_q_01_missing_o : xbsIndex_r4/Gateway Out  inherit_from_input=on  hdl_port=on  timing_constraint=Data Rate  locs_specified=off  LOCs={}  UseAsDAC=off  DACChannel='1'  block_type=gatewayout
      settings: infoedit="Gateway out block.  Converts Xilinx fixed-point or floating-point type inputs into ouputs of type Simulink integer, single, double, or fixed point.<br><br>Hardware notes:  In hardware these blocks become top level output ports or are discarded, depending on how they are configured."
  tbt_poly_q_scope : Scope  NumInputPorts=2
      settings: TimeRange=0.00011214  YMin=-0.1~-1.5  YMax=1~1.5  SaveName=ScopeData11  MaxDataPoints=1000000  SampleInput=on
  tbt_poly_q_scope1 : Scope  NumInputPorts=3
      settings: TimeRange=0.00011214  YMin=-0.1~-1.5~-5  YMax=1~1.5~5  SaveName=ScopeData12  MaxDataPoints=1000000  SampleInput=on
  tbt_poly_q_scope2 : Scope  NumInputPorts=2
      settings: TimeRange=0.00018  YMin=-5.05447e-005~0.9999999998750002  YMax=-5.05447e-005~1.000000000125  SaveName=ScopeData17  MaxDataPoints=1000000  SampleInput=on
  Q_out : Outport
  I_out : Outport  Port=2
  valid_out : Outport  Port=3
  ch_out : Outport  Port=4
  wires:
  I_in/1 -> cic_fofb_i/1, Gateway Out5/1
  Q_in/1 -> cic_fofb_q/1, Gateway Out4/1
  Relational2/1 -> cic_fofb_q/2, cic_fofb_i/2, Gateway Out6/1
  ch_in/1 -> Relational2/1
  cic_fofb_i/6 -> Delay/1
  cic_fofb_i/1 -> Terminator/1
  cic_fofb_i/4 -> Terminator1/1
  cic_fofb_i/5 -> Terminator2/1
  cic_fofb_i/7 -> Terminator3/1
  cic_fofb_q/1 -> Terminator5/1
  cic_fofb_q/4 -> Terminator6/1
  cic_fofb_q/5 -> Terminator7/1
  cic_fofb_q/6 -> Terminator8/1
  cic_fofb_q/7 -> Terminator9/1
  Constant1/1 -> Relational2/2
  Reg/1(dout) -> Q_out/1
  cic_fofb_q/3 -> Reg/1(din)
  cic_fofb_q/2 -> Reg/2(en)
  Reg1/1(dout) -> I_out/1, Gateway Out3/1
  cic_fofb_i/3 -> Reg1/1(din)
  cic_fofb_i/2 -> Reg1/2(en)
  Reg1/2(valid_out) -> valid_out/1
  Delay/1 -> ch_out/1, Gateway Out2/1
  Reg/2(valid_out) -> Terminator11/1
  cic_fofb_q/8 -> cic_fofb_q_01_missing_o/1
  cic_fofb_i/8 -> Gateway Out1/1
  cic_fofb_q_01_missing_o/1 -> tbt_poly_q_scope/1
  Gateway Out1/1 -> tbt_poly_q_scope/2
  Gateway Out2/1 -> tbt_poly_q_scope2/2
  Gateway Out3/1 -> tbt_poly_q_scope2/1
  Gateway Out4/1 -> tbt_poly_q_scope1/1
  Gateway Out5/1 -> tbt_poly_q_scope1/2
  Gateway Out6/1 -> tbt_poly_q_scope1/3

== system ddc_bpm_476_066/FOFB_amp/fofb_amp1/FOFB_CORDIC/TDDM_fofb_cordic1 ==
  fofb_cordic_din : Inport
  fofb_cordic_pin : Inport  Port=2
  fofb_cordic_ch_in : Inport  Port=3
  TDDM_fofb_cordic1_int : Subsystem
  TDDM_tbt_cordic1 : Subsystem
  Terminator : Terminator
  Terminator1 : Terminator
  fofb_cordic_data0_out : Outport
  fofb_cordic_data1_out : Outport  Port=2
  fofb_cordic_phase0_out : Outport  Port=3
  fofb_cordic_phase1_out : Outport  Port=4
  wires:
  TDDM_fofb_cordic1_int/2(dout_ch1) -> fofb_cordic_data1_out/1
  fofb_cordic_din/1 -> TDDM_fofb_cordic1_int/1(din)
  fofb_cordic_ch_in/1 -> TDDM_fofb_cordic1_int/2(ch_in), TDDM_tbt_cordic1/2(ch_in)
  TDDM_fofb_cordic1_int/1(dout_ch0) -> fofb_cordic_data0_out/1
  TDDM_fofb_cordic1_int/3(ch_out) -> Terminator/1
  TDDM_tbt_cordic1/2(dout_ch1) -> fofb_cordic_phase1_out/1
  fofb_cordic_pin/1 -> TDDM_tbt_cordic1/1(din)
  TDDM_tbt_cordic1/1(dout_ch0) -> fofb_cordic_phase0_out/1
  TDDM_tbt_cordic1/3(ch_out) -> Terminator1/1

== system ddc_bpm_476_066/FOFB_amp/fofb_amp1/FOFB_amp/Reg ==
  din : Inport
  Convert : xbsIndex_r4/Convert  gui_display_data_type=Fixed-point  arith_type="Signed  (2's comp)"  n_bits=24  bin_pt=22  float_type=Single  exp_bits=8  fraction_bits=24  quantization="Round  (unbiased: +/- Inf)"  overflow=Flag as error  en=off  latency=0  dbl_ovrd=off  pipeline=off  block_type=convert
  Register : xbsIndex_r4/Register  init=0  rst=off  en=off  dbl_ovrd=off  block_type=register
      settings: xl_area=[0, 0, 0, 0, 0, 0, 0]  block_version=VER_STRING_GOES_HERE
  Reinterpret2 : xbsIndex_r4/Reinterpret  force_arith_type=on  arith_type="Signed  (2's comp)"  force_bin_pt=on  bin_pt=23  block_type=cast
      settings: block_version=VER_STRING_GOES_HERE
  dout : Outport
  wires:
  Register/1 -> dout/1
  din/1 -> Reinterpret2/1
  Reinterpret2/1 -> Convert/1
  Convert/1 -> Register/1

== system ddc_bpm_476_066/FOFB_amp/fofb_amp1/FOFB_amp/Reg1 ==
  din : Inport
  Convert : xbsIndex_r4/Convert  gui_display_data_type=Fixed-point  arith_type="Signed  (2's comp)"  n_bits=24  bin_pt=22  float_type=Single  exp_bits=8  fraction_bits=24  quantization="Round  (unbiased: +/- Inf)"  overflow=Flag as error  en=off  latency=0  dbl_ovrd=off  pipeline=off  block_type=convert
  Register : xbsIndex_r4/Register  init=0  rst=off  en=off  dbl_ovrd=off  block_type=register
      settings: xl_area=[0, 0, 0, 0, 0, 0, 0]  block_version=VER_STRING_GOES_HERE
  Reinterpret2 : xbsIndex_r4/Reinterpret  force_arith_type=on  arith_type="Signed  (2's comp)"  force_bin_pt=on  bin_pt=23  block_type=cast
      settings: block_version=VER_STRING_GOES_HERE
  dout : Outport
  wires:
  Register/1 -> dout/1
  din/1 -> Reinterpret2/1
  Reinterpret2/1 -> Convert/1
  Convert/1 -> Register/1
